simulink model "chap02_111"  (R2020a)
settings: Solver=VariableStepAuto  StartTime=0.0  StopTime=10.0  RelTol=1e-3
settings Model: Creator=chen_w3  LastModifiedBy=chen_w3

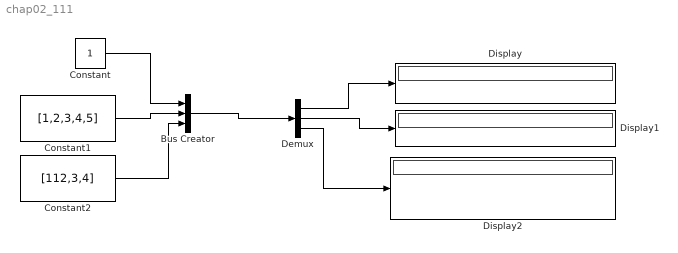
== system chap02_111 ==
  Bus Creator : BusCreator  Inputs=3
  Constant : Constant
  Constant1 : Constant  Value=[1,2,3,4,5]
  Constant2 : Constant  Value=[112,3,4]
  Demux : Demux  Outputs={1,5,3}  BusSelectionMode=on
      settings: DisplayOption=none
  Display : Display
  Display1 : Display
  Display2 : Display
  wires:
  Demux/1 -> Display/1
  Demux/2 -> Display1/1
  Demux/3 -> Display2/1
  Bus Creator/1 -> Demux/1
  Constant/1 -> Bus Creator/1
  Constant1/1 -> Bus Creator/2
  Constant2/1 -> Bus Creator/3
